simulink model "Control_digital_simu"  (R2021a)
settings: Solver=VariableStepAuto  StartTime=0.0  StopTime=2.0  RelTol=1e-3
settings Model: Creator=mogic  LastModifiedBy=mogic

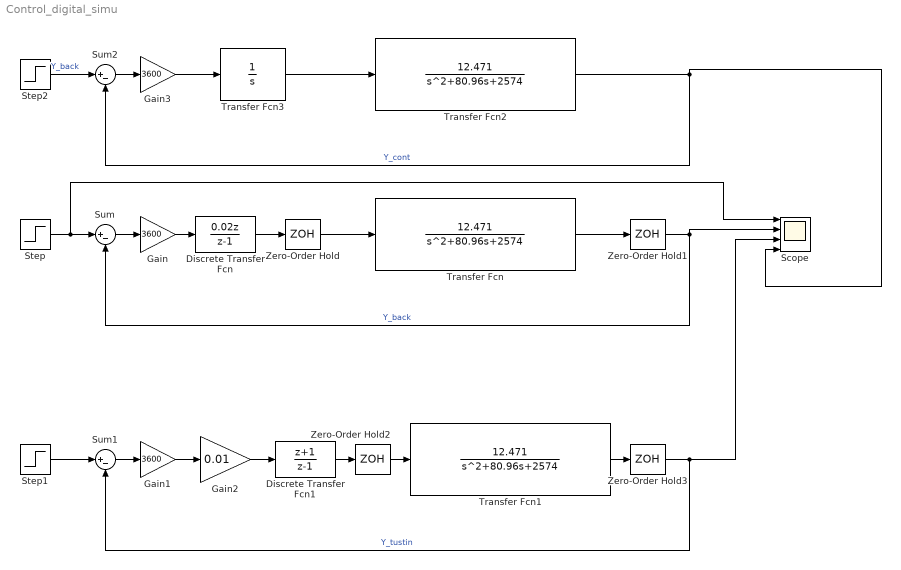
== system Control_digital_simu ==
  Discrete Transfer Fcn : DiscreteTransferFcn  Numerator=[0.02 0]  Denominator=[1 -1]
  Discrete Transfer Fcn1 : DiscreteTransferFcn  Numerator=[1 1]  Denominator=[1 -1]
  Gain : Gain  Gain=3600
  Gain1 : Gain  Gain=3600
  Gain2 : Gain  Gain=0.01
  Gain3 : Gain  Gain=3600
  Scope : Scope  NumInputPorts=4
  Step : Step  SampleTime=0.02
  Step1 : Step  SampleTime=0.02
  Step2 : Step  SampleTime=0.02
  Sum : Sum  Inputs=|+-
  Sum1 : Sum  Inputs=|+-
  Sum2 : Sum  Inputs=|+-
  Transfer Fcn : TransferFcn  Numerator=[12.471]  Denominator=[1 80.96 2574]
  Transfer Fcn1 : TransferFcn  Numerator=[12.471]  Denominator=[1 80.96 2574]
  Transfer Fcn2 : TransferFcn  Numerator=[12.471]  Denominator=[1 80.96 2574]
  Transfer Fcn3 : TransferFcn  Denominator=[1 0]
  Zero-Order Hold{,1..3} (4 alike) : ZeroOrderHold  SampleTime=0.02
  wires:
  Zero-Order Hold/1 -> Transfer Fcn/1
  Step/1 -> Scope/1, Sum/1
  Sum/1 -> Gain/1
  Transfer Fcn/1 -> Zero-Order Hold1/1
  Zero-Order Hold1/1 -> Scope/2, Sum/2  "Y_back"
  Discrete Transfer Fcn/1 -> Zero-Order Hold/1
  Gain/1 -> Discrete Transfer Fcn/1
  Zero-Order Hold3/1 -> Scope/3, Sum1/2  "Y_tustin"
  Transfer Fcn1/1 -> Zero-Order Hold3/1
  Step1/1 -> Sum1/1
  Sum1/1 -> Gain1/1
  Discrete Transfer Fcn1/1 -> Zero-Order Hold2/1
  Zero-Order Hold2/1 -> Transfer Fcn1/1
  Gain1/1 -> Gain2/1
  Gain2/1 -> Discrete Transfer Fcn1/1
  Transfer Fcn2/1 -> Scope/4, Sum2/2  "Y_cont"
  Step2/1 -> Sum2/1  "Y_back"
  Sum2/1 -> Gain3/1
  Transfer Fcn3/1 -> Transfer Fcn2/1
  Gain3/1 -> Transfer Fcn3/1
